simulink model "untitled"  (R2019a)
settings: Solver=ode4  StartTime=0.0  StopTime=50  FixedStep=0.01  RelTol=1e-3
settings Model: Creator=Админ  LastModifiedBy=Sozonov_AA
settings SolverCC: AlgebraicLoopSolver=LineSearch

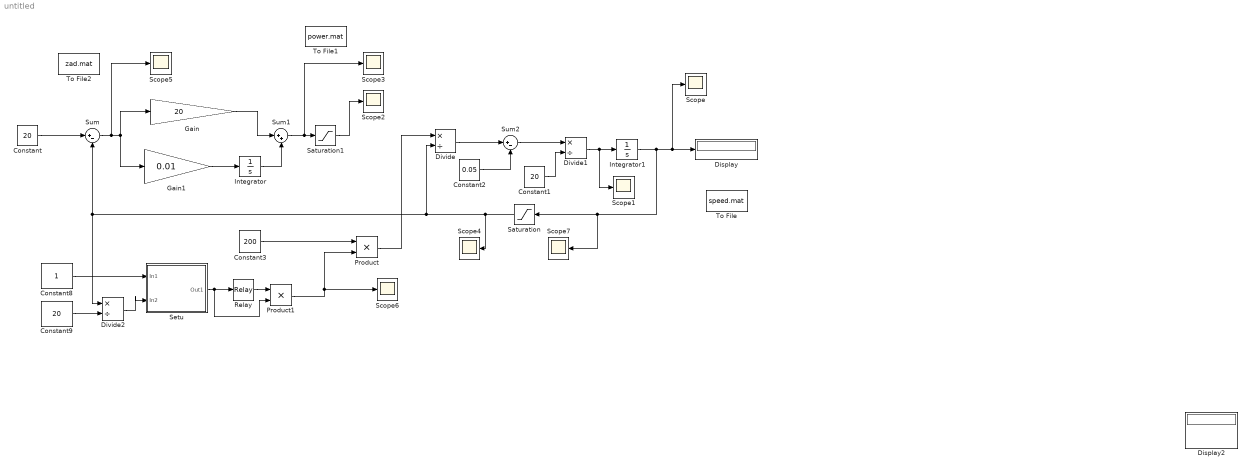
== system untitled ==
  Constant : Constant  Value=20
  Constant1 : Constant  Value=20
  Constant2 : Constant  Value=0.05
  Constant3 : Constant  Value=200  VectorParams1D=off
  Constant8 : Constant  VectorParams1D=off
  Constant9 : Constant  Value=20  VectorParams1D=off
  Display : Display
  Display2 : Display
  Divide : Product  Inputs=*/
  Divide1 : Product  Inputs=*/
  Divide2 : Product  Inputs=*/
  Gain : Gain  Gain=20
  Gain1 : Gain  Gain=0.01
  Integrator : Integrator
  Integrator1 : Integrator
  Product : Product
  Product1 : Product
  Relay : Relay  OnSwitchValue=0.025  OffSwitchValue=0.02
  Saturation : Saturate  UpperLimit=10000  LowerLimit=0.01
  Saturation1 : Saturate  UpperLimit=200  LowerLimit=0
  Scope{,1..7} (8 alike) : Scope
  Setu : Subsystem
  Sum : Sum  Inputs=|+-
  Sum1 : Sum  Inputs=|++
  Sum2 : Sum  Inputs=|+-
  To File : ToFile  Filename=speed.mat  MatrixName=sped  SaveFormat=Timeseries
  To File1 : ToFile  Filename=power.mat  MatrixName=power  SaveFormat=Timeseries
  To File2 : ToFile  Filename=zad.mat  MatrixName=zad  SaveFormat=Timeseries
  wires:
  Constant/1 -> Sum/1
  Sum/1 -> Scope5/1, Gain1/1, Gain/1
  Gain1/1 -> Integrator/1
  Gain/1 -> Sum1/1
  Integrator/1 -> Sum1/2
  Sum1/1 -> Saturation1/1, Scope3/1
  Divide/1 -> Sum2/1
  Sum2/1 -> Divide1/1
  Constant2/1 -> Sum2/2
  Constant1/1 -> Divide1/2
  Integrator1/1 -> Scope7/1, Saturation/1, Scope/1, Display/1
  Divide1/1 -> Scope1/1, Integrator1/1
  Saturation/1 -> Scope4/1, Divide/2, Divide2/1, Sum/2
  Constant8/1 -> Setu/1(In1)
  Constant9/1 -> Divide2/2
  Setu/1(Out1) -> Product1/2, Relay/1
  Divide2/1 -> Setu/2(In2)
  Product/1 -> Divide/1
  Constant3/1 -> Product/1
  Saturation1/1 -> Scope2/1
  Relay/1 -> Product1/1
  Product1/1 -> Scope6/1, Product/2

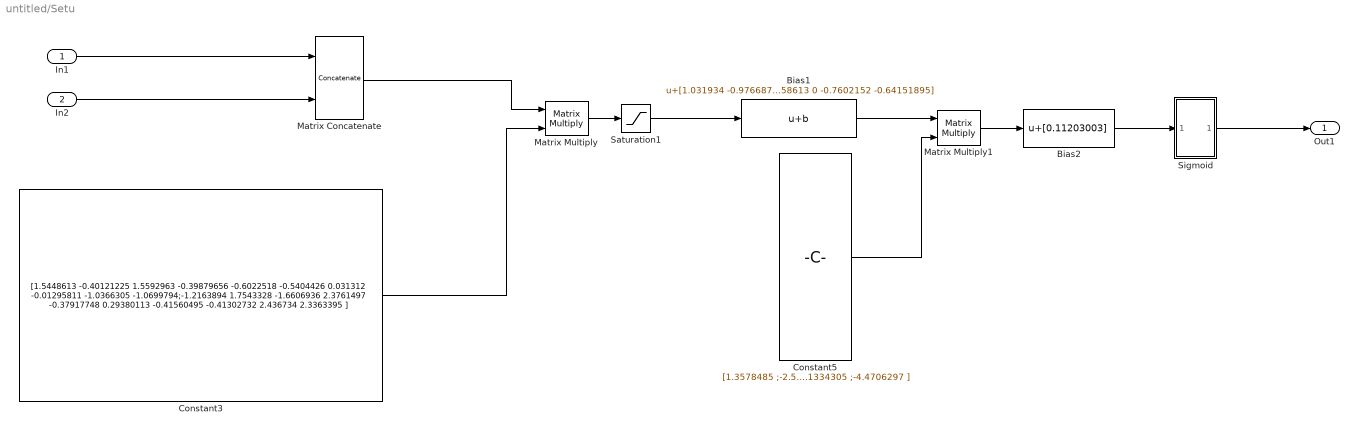
== system untitled/Setu ==
  In1 : Inport
  In2 : Inport  Port=2
  Bias1 : Bias  Bias=[1.031934 -0.97668713 0.9861093 -1.074624 0 0 -0.02858613 0 -0.7602152 -0.64151895]
  Bias2 : Bias  Bias=[0.11203003]
  Constant3 : Constant  Value=[1.5448613 -0.40121225 1.5592963 -0.39879656 -0.6022518 -0.5404426 0.031312 -0.01295811 -1.0366305 -1.0699794;-1.2163894 1.7543328 -1.6606936 2.3761497 -0.37917748 0.29380113 -0.41560495 -0.41302732 2.436734 2.3363395 ]  VectorParams1D=off
  Constant5 : Constant  Value=|  VectorParams1D=off
      | [1.3578485 ;-2.5840182 ; 3.3212507 ;-2.2377758 ; 0.02387977;-0.3912089 ;-0.2691364;
      | -0.45223475;-4.1334305 ;-4.4706297 ]
  Matrix Concatenate : Concatenate  Mode=Multidimensional array  ConcatenateDimension=2
  Matrix Multiply : Product  Multiplication=Matrix(*)
  Matrix Multiply1 : Product  Multiplication=Matrix(*)
  Saturation1 : Saturate  UpperLimit=20  LowerLimit=0
  "Sigmoid " : Subsystem
  Out1 : Outport
  wires:
  Saturation1/1 -> Bias1/1
  Matrix Concatenate/1 -> Matrix Multiply/1
  Matrix Multiply/1 -> Saturation1/1
  In1/1 -> Matrix Concatenate/1
  Matrix Multiply1/1 -> Bias2/1
  Bias1/1 -> Matrix Multiply1/1
  Bias2/1 -> "Sigmoid "/1(In1)
  Constant5/1 -> Matrix Multiply1/2
  Constant3/1 -> Matrix Multiply/2
  "Sigmoid "/1(Out1) -> Out1/1
  In2/1 -> Matrix Concatenate/2

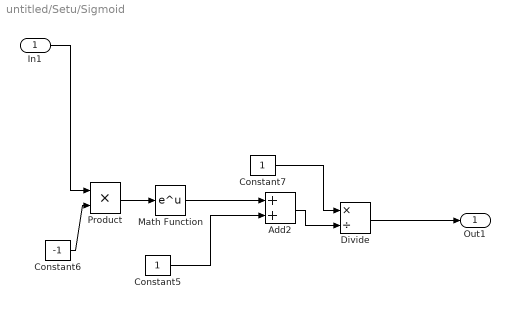
== system untitled/Setu/Sigmoid  ==
  In1 : Inport
  Add2 : Sum
  Constant5 : Constant  VectorParams1D=off
  Constant6 : Constant  Value=-1  VectorParams1D=off
  Constant7 : Constant  VectorParams1D=off
  Divide : Product  Inputs=*/
  Math Function : Math  SaturateOnIntegerOverflow=on
  Product : Product
  Out1 : Outport
  wires:
  Product/1 -> Math Function/1
  Math Function/1 -> Add2/1
  Constant5/1 -> Add2/2
  Constant7/1 -> Divide/1
  Constant6/1 -> Product/2
  In1/1 -> Product/1
  Add2/1 -> Divide/2
  Divide/1 -> Out1/1
